simulink subsystem "Power_Gain2022"  (R2022b)
settings: Solver=VariableStepAuto  StartTime=0.0  StopTime=10.0  RelTol=1e-3
model mask{Kpa=7.3}
  mask prompts: Kpa "Amp"
settings Model: Creator=mrrom  LastModifiedBy=romav
settings OptimizationCC: ReuseModelBlockBuffer=on

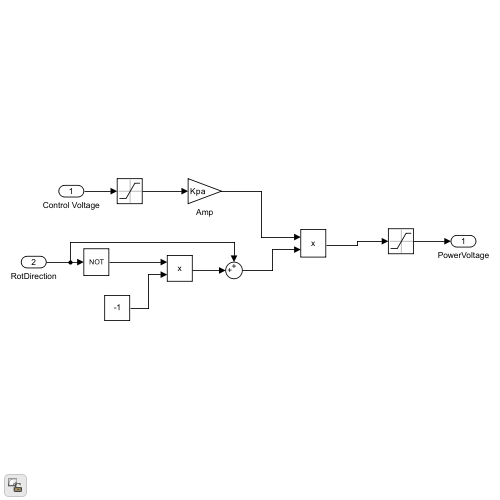
[thumbnail: Simulink's stored preview of the top-level diagram]
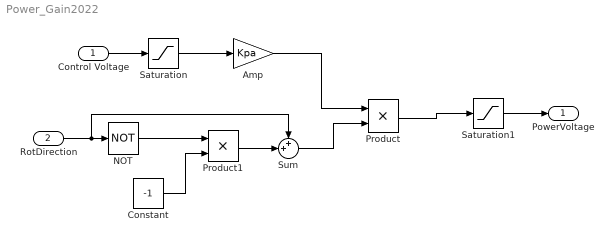
== system Power_Gain2022 ==
  Control Voltage : Inport
  RotDirection : Inport  Port=2
  Amp : Gain  Gain=Kpa
  Constant : Constant  Value=-1
  NOT : Logic  Operator=NOT  AllPortsSameDT=off  OutDataTypeStr=boolean
  Product : Product
  Product1 : Product
  Saturation : Saturate  UpperLimit=3.3  LowerLimit=0
  Saturation1 : Saturate  UpperLimit=24  LowerLimit=-24
  Sum : Sum  Inputs=++|
  PowerVoltage : Outport
  wires:
  Product1/1 -> Sum/2
  Sum/1 -> Product/2
  RotDirection/1 -> NOT/1, Sum/1
  Product/1 -> Saturation1/1
  NOT/1 -> Product1/1
  Amp/1 -> Product/1
  Saturation/1 -> Amp/1
  Constant/1 -> Product1/2
  Control Voltage/1 -> Saturation/1
  Saturation1/1 -> PowerVoltage/1
